simulink model "SWC_FDC_type"  (R2021b)
settings: Solver=FixedStepDiscrete  StartTime=0.0  StopTime=10.0  FixedStep=0.001  RelTol=1e-3
values from neighbouring files (symbols this model uses):
  DID_VCUKey = uint16(0x0202)    [vcu_local_hdr.m]
  DID_XWD = uint16(513)    [vcu_local_hdr.m]
  DIDLen_APSFunConfig = uint16(16)    [vcu_local_hdr.m]
  DIDLen_AutoLock = uint16(1)    [vcu_local_hdr.m]
  DIDLen_DKCKey = uint16(8)    [vcu_local_hdr.m]
  DIDLen_DRLDis = uint16(1)    [vcu_local_hdr.m]
  DIDLen_DynoMode = uint16(1)    [vcu_local_hdr.m]
  DIDLen_FMHTimer = uint16(1)    [vcu_local_hdr.m]
  DIDLen_LFLowPresThre = uint16(1)    [vcu_local_hdr.m]
  DIDLen_LFSensorID = uint16(4)    [vcu_local_hdr.m]
  DIDLen_LRLowPresThre = uint16(1)    [vcu_local_hdr.m]
  DIDLen_LRSensorID = uint16(4)    [vcu_local_hdr.m]
  DIDLen_RFLowPresThre = uint16(1)    [vcu_local_hdr.m]
  DIDLen_RFSensorID = uint16(4)    [vcu_local_hdr.m]
  DIDLen_RRLowPresThre = uint16(1)    [vcu_local_hdr.m]
  DIDLen_RRSensorID = uint16(4)    [vcu_local_hdr.m]
  DIDLen_SensorMode = uint16(1)    [vcu_local_hdr.m]
  DIDLen_TireSize = uint16(16)    [vcu_local_hdr.m]
  DIDLen_TPMSLearnSta = uint16(1)    [vcu_local_hdr.m]
  DIDLen_TurnLampFLThreCurr = uint16(1)    [vcu_local_hdr.m]
  DIDLen_TurnLampFRThreCurr = uint16(1)    [vcu_local_hdr.m]
  DIDLen_TurnLampRLThreCurr = uint16(1)    [vcu_local_hdr.m]
  DIDLen_TurnLampRRThreCurr = uint16(1)    [vcu_local_hdr.m]
  DIDLen_USSConfig = uint16(16)    [vcu_local_hdr.m]
  DIDLen_WhlPres = uint16(4)    [vcu_local_hdr.m]
  DIDLen_WhlSensorBattSta = uint16(1)    [vcu_local_hdr.m]
  DIDLen_WhlTmp = uint16(4)    [vcu_local_hdr.m]
  DIDLen_XWDMode = uint16(1)    [vcu_local_hdr.m]
  DIDNum_APSFunConfig = uint16(0x0903)    [vcu_local_hdr.m]
  DIDNum_AutoLock = uint16(0x0306)    [vcu_local_hdr.m]
  DIDNum_DKCKey = uint16(0x0202)    [vcu_local_hdr.m]
  DIDNum_DRLDis = uint16(0x0307)    [vcu_local_hdr.m]
  DIDNum_DynoMode = uint16(0x0203)    [vcu_local_hdr.m]
  DIDNum_FMHTimer = uint16(0x0305)    [vcu_local_hdr.m]
  DIDNum_LFLowPresThre = uint16(0x0B08)    [vcu_local_hdr.m]
  DIDNum_LFSensorID = uint16(0x0B01)    [vcu_local_hdr.m]
  DIDNum_LRLowPresThre = uint16(0x0B0A)    [vcu_local_hdr.m]
  DIDNum_LRSensorID = uint16(0x0B03)    [vcu_local_hdr.m]
  DIDNum_RFLowPresThre = uint16(0x0B09)    [vcu_local_hdr.m]
  DIDNum_RFSensorID = uint16(0x0B02)    [vcu_local_hdr.m]
  DIDNum_RRLowPresThre = uint16(0x0B0B)    [vcu_local_hdr.m]
  DIDNum_RRSensorID = uint16(0x0B04)    [vcu_local_hdr.m]
  DIDNum_SensorMode = uint16(0x0B0C)    [vcu_local_hdr.m]
  DIDNum_TireSize = uint16(0x0902)    [vcu_local_hdr.m]
  DIDNum_TPMSLearnSta = uint16(0x0B0D)    [vcu_local_hdr.m]
  DIDNum_TurnLampFLThreCurr = uint16(0x0303)    [vcu_local_hdr.m]
  DIDNum_TurnLampFRThreCurr = uint16(0x0301)    [vcu_local_hdr.m]
  DIDNum_TurnLampRLThreCurr = uint16(0x0304)    [vcu_local_hdr.m]
  DIDNum_TurnLampRRThreCurr = uint16(0x0302)    [vcu_local_hdr.m]
  DIDNum_USSConfig = uint16(0x0901)    [vcu_local_hdr.m]
  DIDNum_WhlPres = uint16(0x0B05)    [vcu_local_hdr.m]
  DIDNum_WhlSensorBattSta = uint16(0x0B07)    [vcu_local_hdr.m]
  DIDNum_WhlTmp = uint16(0x0B06)    [vcu_local_hdr.m]
  DIDNum_XWDMode = uint16(0x0201)    [vcu_local_hdr.m]
  DIDVCUKeyLength = uint16(8)    [vcu_local_hdr.m]
  ENUM_DRIVETRAIN_AWD = uint8(  2  )    [vcu_local_hdr.m]
  ENUM_DRIVETRAIN_FWD = uint8(  1  )    [vcu_local_hdr.m]
  ENUM_DRIVETRAIN_RWD = uint8(  0  )    [vcu_local_hdr.m]
  ENUM_REGENLEVEL_INVALID = uint8(  7  )    [vcu_local_hdr.m]
  ENUM_REGENLEVEL_LV1 = uint8(  1  )    [vcu_local_hdr.m]
  ENUM_REGENLEVEL_LV2 = uint8(  2  )    [vcu_local_hdr.m]
  ENUM_REGENLEVEL_LV3 = uint8(  3  )    [vcu_local_hdr.m]
  ENUM_REGENLEVEL_LV4 = uint8(  4  )    [vcu_local_hdr.m]
  ENUM_REGENLEVEL_LV5 = uint8(  5  )    [vcu_local_hdr.m]
  ENUM_REGENLEVEL_OFF = uint8(  0  )    [vcu_local_hdr.m]
  ENUM_REGENLEVEL_OPD = uint8(  6  )    [vcu_local_hdr.m]
  ENUM_TPMSLearnStatus_LEARNED = uint8(  1  )    [vcu_local_hdr.m]
  ENUM_TPMSLearnStatus_LEARNFAIL = uint8(  2  )    [vcu_local_hdr.m]
  ENUM_TPMSLearnStatus_NOTLEARN = uint8(  0  )    [vcu_local_hdr.m]
  ENUM_TPMSSTA_FAT = uint8(  8  )    [vcu_local_hdr.m]
  ENUM_TPMSSTA_LOWBATTERY = uint8(  2  )    [vcu_local_hdr.m]
  FALSE = boolean( 0 )    [vcu_local_hdr.m]
  ONE_INT = uint8(1)    [vcu_local_hdr.m]
  P_boolean = 0.0    [APPTypes.sldd]
  TRUE = boolean( 1 )    [vcu_local_hdr.m]
  ZERO_FLOAT = single(0)    [vcu_local_hdr.m]
  ZERO_INT = uint8(0)    [vcu_local_hdr.m]
undefined symbols (not defined in the file or in its folder): f32_ApsOutVehSpdSig, KHAL_DKCDecryptEnable_flg_ovrdflg, KHAL_DKCDecryptEnable_flg_ovrdval, KHAL_RandomNumberY1_enum, KHAL_RandomNumberY2_enum, KHAL_RandomNumberY_ovrdflg, KHAL_THCMAPTCWarningDTC_flg_ovrdflg, KHAL_THCMAPTCWarningDTC_flg_ovrdval, KHAL_TPMSRESBUTT_flg_ovrdflg, KHAL_TPMSRESBUTT_flg_ovrdval, R_DIDWriteCDD_CSOP_DIDSet_APSFunConfig, R_DIDWriteCDD_CSOP_DIDSet_AutoLock, R_DIDWriteCDD_CSOP_DIDSet_DKCKey, R_DIDWriteCDD_CSOP_DIDSet_DRLDis, R_DIDWriteCDD_CSOP_DIDSet_DynoMode, R_DIDWriteCDD_CSOP_DIDSet_FMHTimer, R_DIDWriteCDD_CSOP_DIDSet_LFLowPresThre, R_DIDWriteCDD_CSOP_DIDSet_LFSensorID, R_DIDWriteCDD_CSOP_DIDSet_LRLowPresThre, R_DIDWriteCDD_CSOP_DIDSet_LRSensorID, R_DIDWriteCDD_CSOP_DIDSet_RFLowPresThre, R_DIDWriteCDD_CSOP_DIDSet_RFSensorID, R_DIDWriteCDD_CSOP_DIDSet_RRLowPresThre, R_DIDWriteCDD_CSOP_DIDSet_RRSensorID, R_DIDWriteCDD_CSOP_DIDSet_SensorMode, R_DIDWriteCDD_CSOP_DIDSet_TireSize, R_DIDWriteCDD_CSOP_DIDSet_TPMSLearnSta, R_DIDWriteCDD_CSOP_DIDSet_TurnLampFLThreCurr, R_DIDWriteCDD_CSOP_DIDSet_TurnLampFRThreCurr, R_DIDWriteCDD_CSOP_DIDSet_TurnLampRLThreCurr, R_DIDWriteCDD_CSOP_DIDSet_TurnLampRRThreCurr, R_DIDWriteCDD_CSOP_DIDSet_USSConfig, R_DIDWriteCDD_CSOP_DIDSet_WhlPres, R_DIDWriteCDD_CSOP_DIDSet_WhlSensorBattSta, R_DIDWriteCDD_CSOP_DIDSet_WhlTmp, R_DIDWriteCDD_CSOP_DIDSet_XWDMode, R_E2E_CAN3_VCU1_CSOP_Write_CAN3_VCU1, R_E2E_CAN3_VCU1_toNIDEC_CSOP_Write_CAN3_VCU1_toNIDEC, R_E2E_CAN4_VCU1_CSOP_Write_CAN4_VCU1, R_FDCCDD_Inner_CSOP_FDC_AppCallSleep, R_HALINCDD_CSOP_PAS_Handler, R_HALINCDD_CSOP_UDS_Main, R_HALOUT_APS_CSOP_ApsOutput, R_HALOUTCDD_CSOP_AppNmStateReq, R_HALOUTCDD_CSOP_SetAcoreRebootCmdACK, R_HALOUTCDD_CSOP_SetSysPwrStat, R_HALOUTCDD_CSOP_SleepRequest, R_IOExpOUT_CDD_CSOP_IOExpSetVal, R_NVMReadCDD_Inner_NVM_ReadOperation, R_NVMWriteCDD_Inner_NVM_WriteOperation, R_UDSCDD_CSOP_DdmRestartOperationCycle, R_WDGCDD_CSOP_Call_Watchdog, R_WDGCDD_CSOP_Call_WDG_AppEnd, R_WDGCDD_CSOP_Call_WDG_AppStart, u16_DIDLen_APSFunConfig, u16_DIDLen_AutoLock, u16_DIDLen_DKCKey, u16_DIDLen_DRLDis, u16_DIDLen_DynoMode, u16_DIDLen_FMHTimer ... (+83)
libraries: simulink x215, FVT_lib x139, hcu_lib x21, hdlsllib x9, app x1, halin x1, halout x1, inp x1, outp x1
(part 11 of 12)

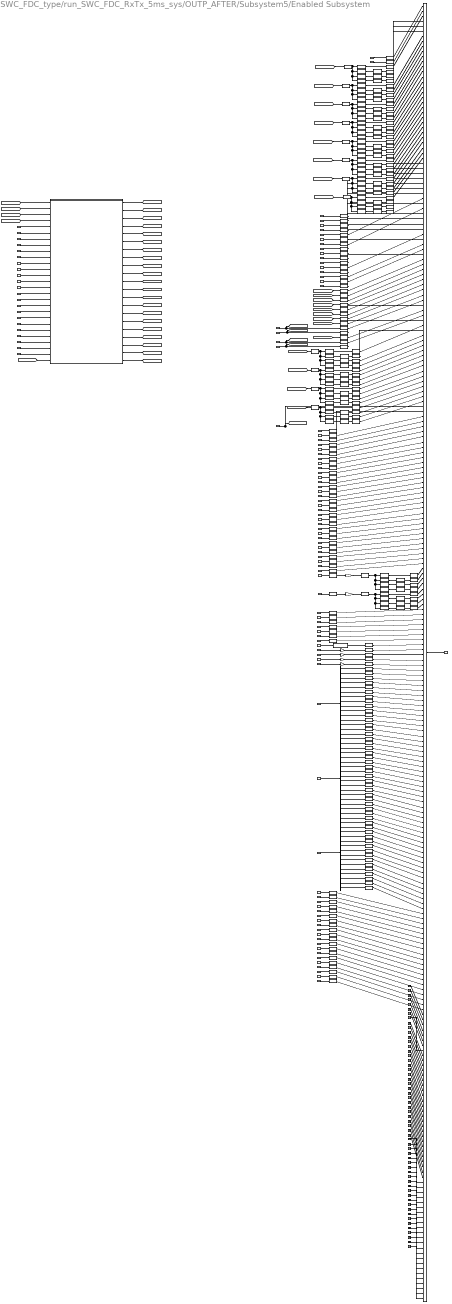
== system SWC_FDC_type/run_SWC_FDC_RxTx_5ms_sys/OUTP_AFTER/Subsystem5/Enabled Subsystem ==
  VOUTP_AntitheftSta_enum : Inport
  VOUTP_DrivetrainSelect_enum : Inport  Port=2
  VOUTP_WriteChkLFID_raw : Inport  Port=3
  VOUTP_WriteChkRFID_raw : Inport  Port=4
  VOUTP_WriteChkLRID_raw : Inport  Port=5
  VOUTP_WriteChkRRID_raw : Inport  Port=6
  VOUTP_WriteChkfinLFID_raw : Inport  Port=7
  VOUTP_WriteChkfinRFID_raw : Inport  Port=8
  VOUTP_WriteChkfinLRID_raw : Inport  Port=9
  VOUTP_WriteChkfinRRID_raw : Inport  Port=10
  VOUTP_LFSensorFail_flg : Inport  Port=11
  VOUTP_RFSensorFail_flg : Inport  Port=12
  VOUTP_LRSensorFail_flg : Inport  Port=13
  VOUTP_RRSensorFail_flg : Inport  Port=14
  VOUTP_LFWheelPSW_raw8 : Inport  Port=15
  VOUTP_RFWheelPSW_raw8 : Inport  Port=16
  VOUTP_LRWheelPSW_raw8 : Inport  Port=17
  VOUTP_RRWheelPSW_raw8 : Inport  Port=18
  VOUTP_LFPindi_enum : Inport  Port=19
  VOUTP_RFPindi_enum : Inport  Port=20
  VOUTP_LRPindi_enum : Inport  Port=21
  VOUTP_RRPindi_enum : Inport  Port=22
  VOUTP_LFP20_raw8 : Inport  Port=23
  VOUTP_RFP20_raw8 : Inport  Port=24
  VOUTP_LRP20_raw8 : Inport  Port=25
  VOUTP_RRP20_raw8 : Inport  Port=26
  VOUTP_LFWheelPress_raw8 : Inport  Port=27
  VOUTP_RFWheelPress_raw8 : Inport  Port=28
  VOUTP_LRWheelPress_raw8 : Inport  Port=29
  VOUTP_RRWheelPress_raw8 : Inport  Port=30
  VOUTP_LFWheelTemp_C : Inport  Port=31
  VOUTP_RFWheelTemp_C : Inport  Port=32
  VOUTP_LRWheelTemp_C : Inport  Port=33
  VOUTP_RRWheelTemp_C : Inport  Port=34
  VOUTP_Flashchkdatavalid_enum : Inport  Port=35
  VOUTP_Flashdatavalid_enum : Inport  Port=36
  VOUTP_unlearnSfali_flg : Inport  Port=37
  VOUTP_unlearnSfailvalid_enum : Inport  Port=38
  VOUTP_Prepresstempvalid_enum : Inport  Port=39
  VOUTP_FlashS1ID_raw : Inport  Port=40
  VOUTP_FlashS2ID_raw : Inport  Port=41
  VOUTP_FlashS3ID_raw : Inport  Port=42
  VOUTP_FlashS41ID_raw : Inport  Port=43
  VOUTP_FlashIDvalid_enum : Inport  Port=44
  VOUTP_ACModeMem_enum : Inport  Port=45
  VOUTP_Face_flg : Inport  Port=46
  VOUTP_Foot_flg : Inport  Port=47
  VOUTP_Frost_flg : Inport  Port=48
  VOUTP_FaceM_flg : Inport  Port=49
  VOUTP_FootM_flg : Inport  Port=50
  VOUTP_CCUSyncSts_flg : Inport  Port=51
  VOUTP_ACForceOFF_flg : Inport  Port=52
  VOUTP_sigRecircSt_flg : Inport  Port=53
  VOUTP_RecAutoFlg_flg : Inport  Port=54
  VOUTP_AirIntenZone1M_enum : Inport  Port=55
  VOUTP_fdefog_flg : Inport  Port=56
  VOUTP_sigSetTempZon1St_C : Inport  Port=57
  VOUTP_sigSetTempZon2StM_C : Inport  Port=58
  VOUT_CountAlarm_enum : Inport  Port=59
  VOUTP_MFSWTri_flg : Inport  Port=60
  VOUTP_MirrorFlodPos_flg : Inport  Port=61
  VOUTP_FuelDoorPos_flg : Inport  Port=62
  VOUTP_LockSetting_flg : Inport  Port=63
  VOUTP_MFRDNBrightReq_pct : Inport  Port=64
  VOUTP_RoomLampMode_flg : Inport  Port=65
  VOUTP_WiperFixMode_flg : Inport  Port=66
  VOUTP_IVIPTGUSStaSW_flg : Inport  Port=67
  VOUTP_EAPS1MIN_pct : Inport  Port=68
  VOUTP_EAPS2MIN_pct : Inport  Port=69
  VOUTP_HoodSW_flg : Inport  Port=70
  VOUTP_TailgateSW_flg : Inport  Port=71
  VOUTP_CTDLockSW_flg : Inport  Port=72
  VOUTP_TailgateHDSW_flg : Inport  Port=73
  VOUTP_APMDoorControlSta_flg : Inport  Port=74
  VOUTP_fUnlockSingle_flg : Inport  Port=75
  VOUTP_SaveRegenMode_enum : Inport  Port=76
  VOUTP_AmbFunENFlash_enum : Inport  Port=77
  VOUTP_AmbWelENFlash_enum : Inport  Port=78
  VOUTP_AmbDimENFlash_enum : Inport  Port=79
  VOUTP_AmbLinkDriStaFlash_enum : Inport  Port=80
  VOUTP_AmbPwrWarnENFlash_enum : Inport  Port=81
  VOUTP_AmbODAENFlash_enum : Inport  Port=82
  VOUTP_AmbColorSta1_enum : Inport  Port=83
  VOUTP_AmbColorSta2_enum : Inport  Port=84
  VOUTP_AmbColorSta3_enum : Inport  Port=85
  VOUTP_AmbColorSta4_enum : Inport  Port=86
  VOUTP_AmbColorSta5_enum : Inport  Port=87
  VOUTP_AmbColorSta7_enum : Inport  Port=88
  VOUTP_AmbBrightnessSta1_enum : Inport  Port=89
  VOUTP_AmbBrightnessSta2_enum : Inport  Port=90
  VOUTP_AmbBrightnessSta3_enum : Inport  Port=91
  VOUTP_AmbBrightnessSta4_enum : Inport  Port=92
  VOUTP_AmbBrightnessSta5_enum : Inport  Port=93
  VOUTP_AmbBrightnessSta7_enum : Inport  Port=94
  BHAL_SYSTPMS_outputs : Inport  Port=95
  VHAL_RandomnumberY_raw1 : Inport  Port=96
  VHAL_RandomnumberY_raw2 : Inport  Port=97
  VHAL_RandomnumberY_raw3 : Inport  Port=98
  VHAL_RandomnumberY_raw4 : Inport  Port=99
  VHAL_RandomnumberY_raw5 : Inport  Port=100
  VHAL_RandomnumberY_raw6 : Inport  Port=101
  VHAL_RandomnumberY_raw7 : Inport  Port=102
  VHAL_RandomnumberY_raw8 : Inport  Port=103
  VHAL_funAuto_flg : Inport  Port=104
  VHAL_DiagDRLOFF_flg : Inport  Port=105
  VHAL_DiagFMHT_s : Inport  Port=106
  VHAL_DiagFLTC_mA : Inport  Port=107
  VHAL_DiagFRTC_mA : Inport  Port=108
  VHAL_DiagRLTC_mA : Inport  Port=109
  VHAL_DiagRRTC_mA : Inport  Port=110
  VHAL_USSConfig_raw8 : Inport  Port=111
  VHAL_TireSize_raw8 : Inport  Port=112
  VHAL_APSFunConfig_raw8 : Inport  Port=113
  Bitwise AND{,4,8,14,16,22,26,30,32,36,40,44,48,52} (14 alike) : simulink/Logic and Bit Operations/Bitwise Operator  logicop=AND  UseBitMask=on  BitMask=bin2dec('00000000000000000000000011111111')  BitMaskRealWorld=Stored Integer
  Bitwise AND{1,5,9,15,17,23,27,31,33,37,41,45,49,53} (14 alike) : simulink/Logic and Bit Operations/Bitwise Operator  logicop=AND  UseBitMask=on  BitMask=bin2dec('00000000000000001111111100000000')  BitMaskRealWorld=Stored Integer
  Bitwise AND{2,6,10,12,18,20,24,28,34,38,42,46,50,54} (14 alike) : simulink/Logic and Bit Operations/Bitwise Operator  logicop=AND  UseBitMask=on  BitMask=bin2dec('00000000111111110000000000000000')  BitMaskRealWorld=Stored Integer
  Bitwise AND{3,7,11,13,19,21,25,29,35,39,43,47,51,55} (14 alike) : simulink/Logic and Bit Operations/Bitwise Operator  logicop=AND  UseBitMask=on  BitMask=bin2dec('11111111000000000000000000000000')  BitMaskRealWorld=Stored Integer
  Data Type Conversion{,1,5..13,15..18,20..23,25..27,29..32,34..37,39..40,42..106,108..111,113..116,118..121,123..126,128..130,132..213} (198 alike) : DataTypeConversion  OutDataTypeStr=uint8
  Data Type Conversion{4,14,19,24,28,33,38,41,107,112,117,122,127,131} (14 alike) : DataTypeConversion  OutDataTypeStr=uint32
  Data Type Conversion2 : DataTypeConversion  OutDataTypeStr=single
  Data Type Conversion3 : DataTypeConversion  OutDataTypeStr=single
  Demux : Demux  Outputs=16
  Demux1 : Demux  Outputs=16
  Demux2 : Demux  Outputs=16
  Gain{,1..3} (4 alike) : Gain  Gain=1/10
  Ground{183..187,196..198,200..247,251} (57 alike) : Ground
  Multiply : Gain  Gain=10000
  Multiply1 : Gain  Gain=10000
  Mux : Mux  Inputs=256
  NVM1 : Subsystem
  Shift Arithmetic{,3,6,9,12,17,20,23..24,27,30,33,36,39} (14 alike) : ArithShift  BitShiftNumber=8  BitShiftDirection=Right
  Shift Arithmetic{1,4,7,10,13..14,18,21,25,28,31,34,37,40} (14 alike) : ArithShift  BitShiftNumber=16  BitShiftDirection=Right
  Shift Arithmetic{2,5,8,11,15..16,19,22,26,29,32,35,38,41} (14 alike) : ArithShift  BitShiftNumber=24  BitShiftDirection=Right
  Subsystem : Subsystem
  HAL_NvmWriteData_raw : Outport
  wires:
  Bitwise AND20/1 -> Shift Arithmetic14/1
  Shift Arithmetic4/1 -> Data Type Conversion12/1
  Data Type Conversion12/1 -> Mux/9
  Data Type Conversion30/1 -> Mux/24
  Shift Arithmetic23/1 -> Data Type Conversion40/1
  Bitwise AND1/1 -> Shift Arithmetic/1
  Bitwise AND11/1 -> Shift Arithmetic8/1
  Data Type Conversion5/1 -> Mux/21
  Bitwise AND17/1 -> Shift Arithmetic12/1
  Data Type Conversion32/1 -> Mux/30
  Data Type Conversion13/1 -> Mux/10
  Shift Arithmetic22/1 -> Data Type Conversion32/1
  Shift Arithmetic17/1 -> Data Type Conversion30/1
  Shift Arithmetic18/1 -> Data Type Conversion7/1
  Data Type Conversion14/1 -> Bitwise AND4/1, Bitwise AND7/1, Bitwise AND6/1, Bitwise AND5/1
  Bitwise AND26/1 -> Data Type Conversion29/1
  Data Type Conversion17/1 -> Mux/13
  Data Type Conversion25/1 -> Mux/15
  Data Type Conversion18/1 -> Mux/14
  Bitwise AND29/1 -> Shift Arithmetic19/1
  Shift Arithmetic8/1 -> Data Type Conversion18/1
  Data Type Conversion39/1 -> Mux/31
  Shift Arithmetic10/1 -> Data Type Conversion22/1
  Data Type Conversion6/1 -> Mux/22
  Bitwise AND28/1 -> Shift Arithmetic18/1
  Shift Arithmetic/1 -> Data Type Conversion9/1
  Data Type Conversion42/1 -> Mux/19
  Data Type Conversion11/1 -> Mux/6
  Shift Arithmetic19/1 -> Data Type Conversion27/1
  Data Type Conversion28/1 -> Bitwise AND26/1, Bitwise AND27/1, Bitwise AND28/1, Bitwise AND29/1
  Bitwise AND19/1 -> Shift Arithmetic22/1
  Bitwise AND27/1 -> Shift Arithmetic17/1
  Bitwise AND3/1 -> Shift Arithmetic2/1
  Data Type Conversion1/1 -> Mux/2
  Data Type Conversion26/1 -> Mux/16
  Bitwise AND23/1 -> Shift Arithmetic23/1
  Shift Arithmetic7/1 -> Data Type Conversion17/1
  Shift Arithmetic21/1 -> Data Type Conversion31/1
  Data Type Conversion8/1 -> Mux/3
  Data Type Conversion/1 -> Mux/1
  Bitwise AND10/1 -> Shift Arithmetic7/1
  Data Type Conversion37/1 -> Mux/34
  Data Type Conversion40/1 -> Mux/32
  Data Type Conversion36/1 -> Mux/33
  Bitwise AND/1 -> Data Type Conversion8/1
  Data Type Conversion20/1 -> Mux/11
  Data Type Conversion16/1 -> Mux/8
  Data Type Conversion21/1 -> Mux/12
  Data Type Conversion9/1 -> Mux/4
  Data Type Conversion10/1 -> Mux/5
  Data Type Conversion31/1 -> Mux/29
  Data Type Conversion15/1 -> Mux/7
  Data Type Conversion34/1 -> Mux/27
  Data Type Conversion35/1 -> Mux/28
  Data Type Conversion27/1 -> Mux/26
  Data Type Conversion29/1 -> Mux/23
  Data Type Conversion7/1 -> Mux/25
  Data Type Conversion22/1 -> Mux/17
  Data Type Conversion23/1 -> Mux/18
  Data Type Conversion43/1 -> Mux/20
  Data Type Conversion33/1 -> Bitwise AND19/1, Bitwise AND18/1, Bitwise AND31/1, Bitwise AND30/1
  Data Type Conversion41/1 -> Bitwise AND25/1, Bitwise AND24/1, Bitwise AND17/1, Bitwise AND16/1
  Bitwise AND30/1 -> Data Type Conversion34/1
  Bitwise AND24/1 -> Shift Arithmetic13/1
  Shift Arithmetic12/1 -> Data Type Conversion43/1
  Bitwise AND25/1 -> Shift Arithmetic16/1
  Bitwise AND18/1 -> Shift Arithmetic21/1
  Shift Arithmetic16/1 -> Data Type Conversion6/1
  Shift Arithmetic15/1 -> Data Type Conversion37/1
  Data Type Conversion38/1 -> Bitwise AND21/1, Bitwise AND20/1, Bitwise AND23/1, Bitwise AND22/1
  Bitwise AND31/1 -> Shift Arithmetic20/1
  Shift Arithmetic9/1 -> Data Type Conversion26/1
  Bitwise AND21/1 -> Shift Arithmetic15/1
  Data Type Conversion24/1 -> Bitwise AND14/1, Bitwise AND13/1, Bitwise AND12/1, Bitwise AND15/1
  Bitwise AND13/1 -> Shift Arithmetic11/1
  Bitwise AND9/1 -> Shift Arithmetic6/1
  Bitwise AND15/1 -> Shift Arithmetic9/1
  Bitwise AND12/1 -> Shift Arithmetic10/1
  Bitwise AND7/1 -> Shift Arithmetic5/1
  Shift Arithmetic2/1 -> Data Type Conversion11/1
  Shift Arithmetic1/1 -> Data Type Conversion10/1
  Data Type Conversion19/1 -> Bitwise AND11/1, Bitwise AND10/1, Bitwise AND9/1, Bitwise AND8/1
  Bitwise AND6/1 -> Shift Arithmetic4/1
  Bitwise AND5/1 -> Shift Arithmetic3/1
  Shift Arithmetic20/1 -> Data Type Conversion35/1
  Shift Arithmetic5/1 -> Data Type Conversion13/1
  Bitwise AND4/1 -> Data Type Conversion15/1
  Shift Arithmetic3/1 -> Data Type Conversion16/1
  Bitwise AND8/1 -> Data Type Conversion20/1
  Bitwise AND22/1 -> Data Type Conversion39/1
  Data Type Conversion4/1 -> Bitwise AND3/1, Bitwise AND2/1, Bitwise AND1/1, Bitwise AND/1
  Bitwise AND2/1 -> Shift Arithmetic1/1
  Shift Arithmetic11/1 -> Data Type Conversion23/1
  Shift Arithmetic14/1 -> Data Type Conversion36/1
  Shift Arithmetic13/1 -> Data Type Conversion5/1
  Bitwise AND14/1 -> Data Type Conversion25/1
  Shift Arithmetic6/1 -> Data Type Conversion21/1
  Bitwise AND16/1 -> Data Type Conversion42/1
  VOUTP_DrivetrainSelect_enum/1 -> Data Type Conversion1/1
  VOUTP_AntitheftSta_enum/1 -> Data Type Conversion/1
  Data Type Conversion66/1 -> Mux/57
  Data Type Conversion67/1 -> Mux/55
  VOUTP_ACModeMem_enum/1 -> Data Type Conversion81/1
  Data Type Conversion57/1 -> Mux/48
  VHAL_RandomnumberY_raw7/1 -> Data Type Conversion79/1
  VHAL_RandomnumberY_raw5/1 -> Data Type Conversion77/1
  VHAL_RandomnumberY_raw6/1 -> Data Type Conversion78/1
  Data Type Conversion72/1 -> Mux/62
  Data Type Conversion69/1 -> Mux/59
  VOUTP_Foot_flg/1 -> Data Type Conversion83/1
  [VHAL_NVMLRWheelPress_raw8] -> Data Type Conversion62/1
  VOUTP_LFSensorFail_flg/1 -> Data Type Conversion47/1
  [VHAL_NVMLFWheelPress_raw8] -> Data Type Conversion63/1
  VHAL_RandomnumberY_raw4/1 -> Data Type Conversion76/1
  VOUTP_Flashchkdatavalid_enum/1 -> [VOUTP_Flashchkdatavalid_enum], Data Type Conversion69/1
  Data Type Conversion63/1 -> Mux/51
  Data Type Conversion68/1 -> Mux/58
  Data Type Conversion51/1 -> Mux/39
  Data Type Conversion53/1 -> Mux/44
  VHAL_RandomnumberY_raw1/1 -> Data Type Conversion75/1
  Data Type Conversion48/1 -> Mux/38
  VOUTP_Face_flg/1 -> Data Type Conversion82/1
  VOUTP_LFP20_raw8/1 -> Data Type Conversion59/1
  VOUTP_CCUSyncSts_flg/1 -> Data Type Conversion87/1
  VHAL_RandomnumberY_raw3/1 -> Data Type Conversion74/1
  [VHAL_NVMRFWheelPress_raw8] -> Data Type Conversion61/1
  Data Type Conversion54/1 -> Mux/45
  Data Type Conversion47/1 -> Mux/35
  [VHAL_NVMunlearnSfali_flg] -> Data Type Conversion71/1
  VOUTP_RecAutoFlg_flg/1 -> Data Type Conversion90/1
  Data Type Conversion61/1 -> Mux/52
  VOUTP_fdefog_flg/1 -> Data Type Conversion92/1
  Data Type Conversion55/1 -> Mux/43
  VOUTP_sigRecircSt_flg/1 -> Data Type Conversion89/1
  Data Type Conversion52/1 -> Mux/42
  Data Type Conversion93/1 -> Mux/63
  Data Type Conversion56/1 -> Mux/46
  VOUTP_RFP20_raw8/1 -> Data Type Conversion57/1
  VOUTP_Prepresstempvalid_enum/1 -> [VOUTP_Prepresstempvalid_enum], Data Type Conversion93/1
  VOUTP_FaceM_flg/1 -> Data Type Conversion85/1
  Data Type Conversion58/1 -> Mux/49
  Data Type Conversion65/1 -> Mux/56
  VOUTP_RRPindi_enum/1 -> Data Type Conversion56/1
  VOUTP_FootM_flg/1 -> Data Type Conversion86/1
  Data Type Conversion50/1 -> Mux/41
  VOUTP_Flashdatavalid_enum/1 -> [VOUTP_Flashdatavalid_enum], Data Type Conversion70/1
  [VHAL_NVMRRWheelPress_raw8] -> Data Type Conversion64/1
  Data Type Conversion70/1 -> Mux/60
  [VHAL_NVMRRWheelTemp_C] -> Data Type Conversion68/1
  [VHAL_NVMLFWheelTemp_C] -> Data Type Conversion67/1
  VOUTP_AirIntenZone1M_enum/1 -> Data Type Conversion91/1
  Data Type Conversion64/1 -> Mux/54
  VOUTP_LRP20_raw8/1 -> Data Type Conversion58/1
  Data Type Conversion71/1 -> Mux/61
  VOUTP_RFPindi_enum/1 -> Data Type Conversion53/1
  VOUTP_RRP20_raw8/1 -> Data Type Conversion60/1
  Data Type Conversion49/1 -> Mux/40
  VOUTP_LRPindi_enum/1 -> Data Type Conversion54/1
  VOUTP_LFPindi_enum/1 -> Data Type Conversion55/1
  [VHAL_NVMLRWheelTemp_C] -> Data Type Conversion66/1
  Data Type Conversion62/1 -> Mux/53
  Data Type Conversion60/1 -> Mux/50
  Data Type Conversion59/1 -> Mux/47
  VOUTP_RRWheelPSW_raw8/1 -> Data Type Conversion52/1
  VHAL_RandomnumberY_raw2/1 -> Data Type Conversion73/1
  VOUTP_LRWheelPSW_raw8/1 -> Data Type Conversion50/1
  VHAL_RandomnumberY_raw8/1 -> Data Type Conversion80/1
  Data Type Conversion45/1 -> Mux/36
  VOUTP_ACForceOFF_flg/1 -> Data Type Conversion88/1
  Data Type Conversion46/1 -> Mux/37
  VOUTP_LFWheelPSW_raw8/1 -> Data Type Conversion51/1
  VOUTP_RRSensorFail_flg/1 -> Data Type Conversion48/1
  VOUTP_LRSensorFail_flg/1 -> Data Type Conversion46/1
  [VHAL_NVMRFWheelTemp_C] -> Data Type Conversion65/1
  VOUTP_RFWheelPSW_raw8/1 -> Data Type Conversion49/1
  VOUTP_RFSensorFail_flg/1 -> Data Type Conversion45/1
  VOUTP_Frost_flg/1 -> Data Type Conversion84/1
  Data Type Conversion134/1 -> Mux/120
  Data Type Conversion135/1 -> Mux/121
  Data Type Conversion136/1 -> Mux/122
  Data Type Conversion137/1 -> Mux/123
  Ground185/1 -> Mux/202
  Ground183/1 -> Mux/200
  Ground184/1 -> Mux/201
  Ground197/1 -> Mux/206
  Ground196/1 -> Mux/205
  Ground187/1 -> Mux/204
  Ground186/1 -> Mux/203
  Ground198/1 -> Mux/207
  Ground211/1 -> Mux/228
  Ground221/1 -> Mux/224
  Ground208/1 -> Mux/225
  Ground220/1 -> Mux/223
  Ground218/1 -> Mux/221
  Ground209/1 -> Mux/226
  Ground216/1 -> Mux/219
  Ground217/1 -> Mux/220
  Ground205/1 -> Mux/214
  Ground215/1 -> Mux/218
  Ground207/1 -> Mux/216
  Ground204/1 -> Mux/213
  Ground206/1 -> Mux/215
  Ground203/1 -> Mux/212
  Ground202/1 -> Mux/211
  Ground200/1 -> Mux/209
  Ground201/1 -> Mux/210
  Ground210/1 -> Mux/227
  Ground225/1 -> Mux/208
  Ground214/1 -> Mux/217
  Ground223/1 -> Mux/232
  Ground222/1 -> Mux/231
  Ground213/1 -> Mux/230
  Ground212/1 -> Mux/229
  Ground224/1 -> Mux/233
  Ground219/1 -> Mux/222
  Ground237/1 -> Mux/254
  Ground247/1 -> Mux/250
  Ground234/1 -> Mux/251
  Ground246/1 -> Mux/249
  Ground244/1 -> Mux/247
  Ground235/1 -> Mux/252
  Ground242/1 -> Mux/245
  Ground243/1 -> Mux/246
  Ground231/1 -> Mux/240
  Ground241/1 -> Mux/244
  Ground233/1 -> Mux/242
  Ground230/1 -> Mux/239
  Ground232/1 -> Mux/241
  Ground229/1 -> Mux/238
  Ground228/1 -> Mux/237
  Ground226/1 -> Mux/235
  Ground227/1 -> Mux/236
  Ground236/1 -> Mux/253
  Ground251/1 -> Mux/234
  Ground240/1 -> Mux/243
  Ground239/1 -> Mux/256
  Ground238/1 -> Mux/255
  Ground245/1 -> Mux/248
  Mux/1 -> HAL_NvmWriteData_raw/1
  NVM1/1(VHAL_NVMWriteChkLFID_raw) -> [VHAL_NVMWriteChkLFID_raw]
  VOUTP_WriteChkRFID_raw/1 -> NVM1/6(VOUTP_WriteChkRFID_raw)
  VOUTP_WriteChkLFID_raw/1 -> NVM1/5(VOUTP_WriteChkLFID_raw)
  VOUTP_WriteChkRRID_raw/1 -> NVM1/8(VOUTP_WriteChkRRID_raw)
  VOUTP_WriteChkLRID_raw/1 -> NVM1/7(VOUTP_WriteChkLRID_raw)
  [VOUTP_unlearnSfailvalid_enum] -> NVM1/3(VOUTP_unlearnSfailvalid_enum)
  [VOUTP_Flashchkdatavalid_enum] -> NVM1/1(VOUTP_Flashchkdatavalid_enum)
  [VOUTP_Prepresstempvalid_enum] -> NVM1/4(VOUTP_Prepresstempvalid_enum)
  [VOUTP_Flashdatavalid_enum] -> NVM1/2(VOUTP_Flashdatavalid_enum)
  VOUTP_unlearnSfailvalid_enum/1 -> Data Type Conversion72/1, [VOUTP_unlearnSfailvalid_enum]
  [VHAL_NVMWriteChkfinRRID_raw] -> Data Type Conversion38/1
  [VHAL_NVMWriteChkfinLRID_raw] -> Data Type Conversion33/1
  [VHAL_NVMWriteChkfinRFID_raw] -> Data Type Conversion28/1
  [VHAL_NVMWriteChkfinLFID_raw] -> Data Type Conversion41/1
  [VHAL_NVMWriteChkRRID_raw] -> Data Type Conversion24/1
  [VHAL_NVMWriteChkLRID_raw] -> Data Type Conversion19/1
  [VHAL_NVMWriteChkRFID_raw] -> Data Type Conversion14/1
  [VHAL_NVMWriteChkLFID_raw] -> Data Type Conversion4/1
  VOUT_CountAlarm_enum/1 -> Data Type Conversion99/1
  VOUTP_FuelDoorPos_flg/1 -> Data Type Conversion96/1
  VOUTP_LockSetting_flg/1 -> Data Type Conversion103/1
  VOUTP_WiperFixMode_flg/1 -> Data Type Conversion104/1
  VOUTP_MFRDNBrightReq_pct/1 -> Data Type Conversion100/1
  VOUTP_IVIPTGUSStaSW_flg/1 -> Data Type Conversion102/1
  VOUTP_RoomLampMode_flg/1 -> Data Type Conversion101/1
  VOUTP_MirrorFlodPos_flg/1 -> Data Type Conversion95/1
  VOUTP_sigSetTempZon2StM_C/1 -> Data Type Conversion98/1
  VOUTP_sigSetTempZon1St_C/1 -> Data Type Conversion97/1
  VOUTP_MFSWTri_flg/1 -> Data Type Conversion94/1
  VOUTP_WriteChkfinLRID_raw/1 -> NVM1/11(VOUTP_WriteChkfinLRID_raw)
  VOUTP_WriteChkfinRRID_raw/1 -> NVM1/12(VOUTP_WriteChkfinRRID_raw)
  VOUTP_WriteChkfinLFID_raw/1 -> NVM1/9(VOUTP_WriteChkfinLFID_raw)
  VOUTP_WriteChkfinRFID_raw/1 -> NVM1/10(VOUTP_WriteChkfinRFID_raw)
  VOUTP_LFWheelPress_raw8/1 -> NVM1/13(VOUTP_LFWheelPress_raw8)
  VOUTP_RFWheelPress_raw8/1 -> NVM1/14(VOUTP_RFWheelPress_raw8)
  VOUTP_RRWheelPress_raw8/1 -> NVM1/16(VOUTP_RRWheelPress_raw8)
  VOUTP_LRWheelPress_raw8/1 -> NVM1/15(VOUTP_LRWheelPress_raw8)
  VOUTP_LFWheelTemp_C/1 -> NVM1/17(VOUTP_LFWheelTemp_C)
  VOUTP_RFWheelTemp_C/1 -> NVM1/18(VOUTP_RFWheelTemp_C)
  VOUTP_LRWheelTemp_C/1 -> NVM1/19(VOUTP_LRWheelTemp_C)
  VOUTP_RRWheelTemp_C/1 -> NVM1/20(VOUTP_RRWheelTemp_C)
  VOUTP_unlearnSfali_flg/1 -> NVM1/21(VOUTP_unlearnSfali_flg)
  BHAL_SYSTPMS_outputs/1 -> NVM1/22(BHAL_SYSTPMS_outputs)
  VOUTP_FlashS41ID_raw/1 -> NVM1/26(VOUTP_FlashS4ID_raw)
  VOUTP_FlashS2ID_raw/1 -> NVM1/24(VOUTP_FlashS2ID_raw)
  VOUTP_FlashS1ID_raw/1 -> NVM1/23(VOUTP_FlashS1ID_raw)
  VOUTP_FlashS3ID_raw/1 -> NVM1/25(VOUTP_FlashS3ID_raw)
  [VOUTP_FlashIDvalid_enum] -> NVM1/27(VOUTP_FlashIDvalid_enum)
  VOUTP_FlashIDvalid_enum/1 -> Mux/80, [VOUTP_FlashIDvalid_enum]
  Shift Arithmetic32/1 -> Data Type Conversion116/1
  Bitwise AND35/1 -> Shift Arithmetic26/1
  Shift Arithmetic29/1 -> Data Type Conversion111/1
  Bitwise AND43/1 -> Shift Arithmetic32/1
  Bitwise AND33/1 -> Shift Arithmetic24/1
  Bitwise AND41/1 -> Shift Arithmetic30/1
  [VHAL_NVMFlashS4ID_raw] -> Data Type Conversion122/1
  Shift Arithmetic24/1 -> Data Type Conversion109/1
  Data Type Conversion107/1 -> Bitwise AND35/1, Bitwise AND34/1, Bitwise AND33/1, Bitwise AND32/1
  Shift Arithmetic33/1 -> Data Type Conversion124/1
  Shift Arithmetic34/1 -> Data Type Conversion120/1
  Data Type Conversion117/1 -> Bitwise AND43/1, Bitwise AND42/1, Bitwise AND41/1, Bitwise AND40/1
  Bitwise AND36/1 -> Data Type Conversion113/1
  Bitwise AND40/1 -> Data Type Conversion118/1
  Shift Arithmetic27/1 -> Data Type Conversion114/1
  Bitwise AND32/1 -> Data Type Conversion108/1
  Bitwise AND37/1 -> Shift Arithmetic27/1
  Data Type Conversion122/1 -> Bitwise AND47/1, Bitwise AND46/1, Bitwise AND45/1, Bitwise AND44/1
  Shift Arithmetic26/1 -> Data Type Conversion106/1
  Data Type Conversion112/1 -> Bitwise AND39/1, Bitwise AND38/1, Bitwise AND37/1, Bitwise AND36/1
  Bitwise AND39/1 -> Shift Arithmetic29/1
  Bitwise AND47/1 -> Shift Arithmetic35/1
  Bitwise AND44/1 -> Data Type Conversion123/1
  Bitwise AND46/1 -> Shift Arithmetic34/1
  [VHAL_NVMFlashS3ID_raw] -> Data Type Conversion117/1
  Shift Arithmetic30/1 -> Data Type Conversion119/1
  Bitwise AND34/1 -> Shift Arithmetic25/1
  Shift Arithmetic28/1 -> Data Type Conversion110/1
  Bitwise AND38/1 -> Shift Arithmetic28/1
  Bitwise AND45/1 -> Shift Arithmetic33/1
  [VHAL_NVMFlashS2ID_raw] -> Data Type Conversion112/1
  Shift Arithmetic25/1 -> Data Type Conversion105/1
  Shift Arithmetic35/1 -> Data Type Conversion121/1
  Shift Arithmetic31/1 -> Data Type Conversion115/1
  Bitwise AND42/1 -> Shift Arithmetic31/1
  [VHAL_NVMFlashS1ID_raw] -> Data Type Conversion107/1
  Data Type Conversion109/1 -> Mux/65
  Data Type Conversion105/1 -> Mux/66
  Data Type Conversion106/1 -> Mux/67
  Data Type Conversion114/1 -> Mux/69
  Data Type Conversion110/1 -> Mux/70
  Data Type Conversion111/1 -> Mux/71
  Data Type Conversion119/1 -> Mux/73
  Data Type Conversion115/1 -> Mux/74
  Data Type Conversion116/1 -> Mux/75
  Data Type Conversion124/1 -> Mux/77
  Data Type Conversion120/1 -> Mux/78
  Data Type Conversion121/1 -> Mux/79
  Data Type Conversion108/1 -> Mux/64
  Data Type Conversion113/1 -> Mux/68
  Data Type Conversion118/1 -> Mux/72
  Data Type Conversion123/1 -> Mux/76
  Data Type Conversion75/1 -> Mux/81
  Data Type Conversion73/1 -> Mux/82
  Data Type Conversion74/1 -> Mux/83
  Data Type Conversion76/1 -> Mux/84
  Data Type Conversion77/1 -> Mux/85
  Data Type Conversion78/1 -> Mux/86
  Data Type Conversion79/1 -> Mux/87
  Data Type Conversion80/1 -> Mux/88
  Data Type Conversion81/1 -> Mux/89
  Data Type Conversion82/1 -> Mux/90
  Data Type Conversion83/1 -> Mux/91
  Data Type Conversion84/1 -> Mux/92
  Data Type Conversion85/1 -> Mux/93
  Data Type Conversion86/1 -> Mux/94
  Data Type Conversion87/1 -> Mux/95
  Data Type Conversion88/1 -> Mux/96
  Data Type Conversion89/1 -> Mux/97
  Data Type Conversion90/1 -> Mux/98
  Data Type Conversion91/1 -> Mux/99
  Data Type Conversion92/1 -> Mux/100
  Data Type Conversion97/1 -> Mux/101
  Data Type Conversion98/1 -> Mux/102
  Data Type Conversion99/1 -> Mux/103
  Data Type Conversion94/1 -> Mux/104
  Data Type Conversion95/1 -> Mux/105
  Data Type Conversion96/1 -> Mux/106
  Data Type Conversion103/1 -> Mux/107
  Data Type Conversion100/1 -> Mux/108
  Data Type Conversion101/1 -> Mux/109
  Data Type Conversion104/1 -> Mux/110
  Data Type Conversion102/1 -> Mux/111
  NVM1/21(VHAL_NVMFlashS4ID_raw) -> [VHAL_NVMFlashS4ID_raw]
  NVM1/2(VHAL_NVMWriteChkRFID_raw) -> [VHAL_NVMWriteChkRFID_raw]
  NVM1/3(VHAL_NVMWriteChkLRID_raw) -> [VHAL_NVMWriteChkLRID_raw]
  NVM1/4(VHAL_NVMWriteChkRRID_raw) -> [VHAL_NVMWriteChkRRID_raw]
  NVM1/5(VHAL_NVMWriteChkfinLFID_raw) -> [VHAL_NVMWriteChkfinLFID_raw]
  NVM1/6(VHAL_NVMWriteChkfinRFID_raw) -> [VHAL_NVMWriteChkfinRFID_raw]
  NVM1/7(VHAL_NVMWriteChkfinLRID_raw) -> [VHAL_NVMWriteChkfinLRID_raw]
  NVM1/8(VHAL_NVMWriteChkfinRRID_raw) -> [VHAL_NVMWriteChkfinRRID_raw]
  NVM1/9(VHAL_NVMunlearnSfali_flg) -> [VHAL_NVMunlearnSfali_flg]
  NVM1/10(VHAL_NVMLFWheelPress_raw8) -> [VHAL_NVMLFWheelPress_raw8]
  NVM1/11(VHAL_NVMRFWheelPress_raw8) -> [VHAL_NVMRFWheelPress_raw8]
  NVM1/12(VHAL_NVMLRWheelPress_raw8) -> [VHAL_NVMLRWheelPress_raw8]
  NVM1/13(VHAL_NVMRRWheelPress_raw8) -> [VHAL_NVMRRWheelPress_raw8]
  NVM1/14(VHAL_NVMLFWheelTemp_C) -> [VHAL_NVMLFWheelTemp_C]
  NVM1/15(VHAL_NVMRFWheelTemp_C) -> [VHAL_NVMRFWheelTemp_C]
  NVM1/16(VHAL_NVMLRWheelTemp_C) -> [VHAL_NVMLRWheelTemp_C]
  NVM1/17(VHAL_NVMRRWheelTemp_C) -> [VHAL_NVMRRWheelTemp_C]
  NVM1/18(VHAL_NVMFlashS1ID_raw) -> [VHAL_NVMFlashS1ID_raw]
  NVM1/19(VHAL_NVMFlashS2ID_raw) -> [VHAL_NVMFlashS2ID_raw]
  NVM1/20(VHAL_NVMFlashS3ID_raw) -> [VHAL_NVMFlashS3ID_raw]
  VOUTP_EAPS1MIN_pct/1 -> Data Type Conversion2/1
  VOUTP_EAPS2MIN_pct/1 -> Data Type Conversion3/1
  Multiply/1 -> Data Type Conversion127/1
  Data Type Conversion126/1 -> Mux/115
  Data Type Conversion129/1 -> Mux/113
  Data Type Conversion125/1 -> Mux/114
  Shift Arithmetic37/1 -> Data Type Conversion125/1
  Shift Arithmetic38/1 -> Data Type Conversion126/1
  Data Type Conversion128/1 -> Mux/112
  Bitwise AND48/1 -> Data Type Conversion128/1
  Bitwise AND49/1 -> Shift Arithmetic36/1
  Data Type Conversion127/1 -> Bitwise AND51/1, Bitwise AND50/1, Bitwise AND49/1, Bitwise AND48/1
  Shift Arithmetic36/1 -> Data Type Conversion129/1
  Bitwise AND51/1 -> Shift Arithmetic38/1
  Bitwise AND50/1 -> Shift Arithmetic37/1
  Data Type Conversion2/1 -> Multiply/1
  Bitwise AND54/1 -> Shift Arithmetic40/1
  Bitwise AND55/1 -> Shift Arithmetic41/1
  Shift Arithmetic39/1 -> Data Type Conversion133/1
  Data Type Conversion131/1 -> Bitwise AND52/1, Bitwise AND53/1, Bitwise AND54/1, Bitwise AND55/1
  Bitwise AND53/1 -> Shift Arithmetic39/1
  Bitwise AND52/1 -> Data Type Conversion132/1
  Shift Arithmetic41/1 -> Data Type Conversion130/1
  Shift Arithmetic40/1 -> Data Type Conversion44/1
  Multiply1/1 -> Data Type Conversion131/1
  Data Type Conversion132/1 -> Mux/116
  Data Type Conversion133/1 -> Mux/117
  Data Type Conversion44/1 -> Mux/118
  Data Type Conversion130/1 -> Mux/119
  Data Type Conversion3/1 -> Multiply1/1
  VOUTP_HoodSW_flg/1 -> Data Type Conversion134/1
  VOUTP_TailgateHDSW_flg/1 -> Data Type Conversion137/1
  VOUTP_CTDLockSW_flg/1 -> Data Type Conversion136/1
  VOUTP_TailgateSW_flg/1 -> Data Type Conversion135/1
  VOUTP_APMDoorControlSta_flg/1 -> Data Type Conversion138/1
  Data Type Conversion138/1 -> Mux/124
  VHAL_funAuto_flg/1 -> Data Type Conversion139/1
  VHAL_DiagDRLOFF_flg/1 -> Data Type Conversion140/1
  Data Type Conversion139/1 -> Mux/125
  Data Type Conversion140/1 -> Mux/126
  Data Type Conversion141/1 -> Mux/127
  Data Type Conversion142/1 -> Mux/128
  Data Type Conversion143/1 -> Mux/129
  Data Type Conversion144/1 -> Mux/130
  Data Type Conversion145/1 -> Mux/131
  Demux/1 -> Data Type Conversion146/1
  Demux/2 -> Data Type Conversion147/1
  Demux/3 -> Data Type Conversion148/1
  Demux/4 -> Data Type Conversion149/1
  Demux/5 -> Data Type Conversion150/1
  Demux/6 -> Data Type Conversion151/1
  Demux/7 -> Data Type Conversion152/1
  Demux/8 -> Data Type Conversion153/1
  VHAL_USSConfig_raw8/1 -> Demux/1
  Data Type Conversion146/1 -> Mux/132
  Data Type Conversion147/1 -> Mux/133
  Data Type Conversion148/1 -> Mux/134
  Data Type Conversion149/1 -> Mux/135
  Data Type Conversion150/1 -> Mux/136
  Data Type Conversion151/1 -> Mux/137
  Data Type Conversion152/1 -> Mux/138
  Data Type Conversion153/1 -> Mux/139
  Demux/16 -> Data Type Conversion161/1
  Demux/15 -> Data Type Conversion160/1
  Demux/14 -> Data Type Conversion159/1
  Demux/13 -> Data Type Conversion158/1
  Demux/12 -> Data Type Conversion157/1
  Demux/11 -> Data Type Conversion156/1
  Demux/10 -> Data Type Conversion155/1
  Demux/9 -> Data Type Conversion154/1
  Data Type Conversion154/1 -> Mux/140
  Data Type Conversion155/1 -> Mux/141
  Data Type Conversion156/1 -> Mux/142
  Data Type Conversion157/1 -> Mux/143
  Data Type Conversion158/1 -> Mux/144
  Data Type Conversion159/1 -> Mux/145
  Data Type Conversion160/1 -> Mux/146
  Data Type Conversion161/1 -> Mux/147
  Data Type Conversion177/1 -> Mux/163
  Data Type Conversion176/1 -> Mux/162
  Data Type Conversion175/1 -> Mux/161
  Data Type Conversion174/1 -> Mux/160
  Data Type Conversion173/1 -> Mux/159
  Data Type Conversion172/1 -> Mux/158
  Data Type Conversion171/1 -> Mux/157
  Data Type Conversion170/1 -> Mux/156
  Demux1/9 -> Data Type Conversion170/1
  Demux1/10 -> Data Type Conversion171/1
  Demux1/11 -> Data Type Conversion172/1
  Demux1/12 -> Data Type Conversion173/1
  Demux1/13 -> Data Type Conversion174/1
  Demux1/14 -> Data Type Conversion175/1
  Demux1/15 -> Data Type Conversion176/1
  Demux1/16 -> Data Type Conversion177/1
  Data Type Conversion169/1 -> Mux/155
  Data Type Conversion168/1 -> Mux/154
  Data Type Conversion167/1 -> Mux/153
  Data Type Conversion166/1 -> Mux/152
  Data Type Conversion165/1 -> Mux/151
  Data Type Conversion164/1 -> Mux/150
  Data Type Conversion163/1 -> Mux/149
  Data Type Conversion162/1 -> Mux/148
  VHAL_TireSize_raw8/1 -> Demux1/1
  Demux1/8 -> Data Type Conversion169/1
  Demux1/7 -> Data Type Conversion168/1
  Demux1/6 -> Data Type Conversion167/1
  Demux1/5 -> Data Type Conversion166/1
  Demux1/4 -> Data Type Conversion165/1
  Demux1/3 -> Data Type Conversion164/1
  Demux1/2 -> Data Type Conversion163/1
  Demux1/1 -> Data Type Conversion162/1
  Demux2/1 -> Data Type Conversion178/1
  Demux2/2 -> Data Type Conversion179/1
  Demux2/3 -> Data Type Conversion180/1
  Demux2/4 -> Data Type Conversion181/1
  Demux2/5 -> Data Type Conversion182/1
  Demux2/6 -> Data Type Conversion183/1
  Demux2/7 -> Data Type Conversion184/1
  Demux2/8 -> Data Type Conversion185/1
  VHAL_APSFunConfig_raw8/1 -> Demux2/1
  Data Type Conversion178/1 -> Mux/164
  Data Type Conversion179/1 -> Mux/165
  Data Type Conversion180/1 -> Mux/166
  Data Type Conversion181/1 -> Mux/167
  Data Type Conversion182/1 -> Mux/168
  Data Type Conversion183/1 -> Mux/169
  Data Type Conversion184/1 -> Mux/170
  Data Type Conversion185/1 -> Mux/171
  Demux2/16 -> Data Type Conversion193/1
  Demux2/15 -> Data Type Conversion192/1
  Demux2/14 -> Data Type Conversion191/1
  Demux2/13 -> Data Type Conversion190/1
  Demux2/12 -> Data Type Conversion189/1
  Demux2/11 -> Data Type Conversion188/1
  Demux2/10 -> Data Type Conversion187/1
  Demux2/9 -> Data Type Conversion186/1
  Data Type Conversion186/1 -> Mux/172
  Data Type Conversion187/1 -> Mux/173
  Data Type Conversion188/1 -> Mux/174
  Data Type Conversion189/1 -> Mux/175
  Data Type Conversion190/1 -> Mux/176
  Data Type Conversion191/1 -> Mux/177
  Data Type Conversion192/1 -> Mux/178
  Data Type Conversion193/1 -> Mux/179
  VOUTP_fUnlockSingle_flg/1 -> Data Type Conversion194/1
  Data Type Conversion194/1 -> Mux/180
  Gain3/1 -> Data Type Conversion145/1
  Gain2/1 -> Data Type Conversion144/1
  Gain1/1 -> Data Type Conversion143/1
  Gain/1 -> Data Type Conversion142/1
  Subsystem/1(Out1) -> Data Type Conversion141/1
  VHAL_DiagFMHT_s/1 -> Subsystem/1(VOUTP_DiagFMHT_s)
  VHAL_DiagFRTC_mA/1 -> Gain1/1
  VHAL_DiagRLTC_mA/1 -> Gain2/1
  VHAL_DiagRRTC_mA/1 -> Gain3/1
  VHAL_DiagFLTC_mA/1 -> Gain/1
  VOUTP_SaveRegenMode_enum/1 -> Data Type Conversion195/1
  Data Type Conversion195/1 -> Mux/181
  Data Type Conversion212/1 -> Mux/198
  VOUTP_AmbPwrWarnENFlash_enum/1 -> Data Type Conversion200/1
  Data Type Conversion197/1 -> Mux/183
  Data Type Conversion199/1 -> Mux/185
  VOUTP_AmbColorSta5_enum/1 -> Data Type Conversion206/1
  VOUTP_AmbBrightnessSta1_enum/1 -> Data Type Conversion208/1
  VOUTP_AmbBrightnessSta3_enum/1 -> Data Type Conversion210/1
  Data Type Conversion213/1 -> Mux/199
  Data Type Conversion196/1 -> Mux/182
  Data Type Conversion202/1 -> Mux/188
  Data Type Conversion200/1 -> Mux/186
  VOUTP_AmbBrightnessSta2_enum/1 -> Data Type Conversion209/1
  Data Type Conversion209/1 -> Mux/195
  Data Type Conversion201/1 -> Mux/187
  VOUTP_AmbColorSta3_enum/1 -> Data Type Conversion204/1
  VOUTP_AmbColorSta1_enum/1 -> Data Type Conversion202/1
  VOUTP_AmbBrightnessSta7_enum/1 -> Data Type Conversion213/1
  VOUTP_AmbColorSta4_enum/1 -> Data Type Conversion205/1
  VOUTP_AmbODAENFlash_enum/1 -> Data Type Conversion201/1
  VOUTP_AmbLinkDriStaFlash_enum/1 -> Data Type Conversion199/1
  VOUTP_AmbFunENFlash_enum/1 -> Data Type Conversion196/1
  Data Type Conversion204/1 -> Mux/190
  Data Type Conversion203/1 -> Mux/189
  VOUTP_AmbDimENFlash_enum/1 -> Data Type Conversion198/1
  VOUTP_AmbColorSta2_enum/1 -> Data Type Conversion203/1
  VOUTP_AmbColorSta7_enum/1 -> Data Type Conversion207/1
  Data Type Conversion208/1 -> Mux/194
  VOUTP_AmbWelENFlash_enum/1 -> Data Type Conversion197/1
  Data Type Conversion205/1 -> Mux/191
  VOUTP_AmbBrightnessSta4_enum/1 -> Data Type Conversion211/1
  Data Type Conversion207/1 -> Mux/193
  Data Type Conversion211/1 -> Mux/197
  Data Type Conversion210/1 -> Mux/196
  Data Type Conversion206/1 -> Mux/192
  VOUTP_AmbBrightnessSta5_enum/1 -> Data Type Conversion212/1
  Data Type Conversion198/1 -> Mux/184

== system SWC_FDC_type/run_SWC_FDC_RxTx_5ms_sys/Subsystem2/DKC2/DKC Decryption and Unpack ==
  DKC_ResultData_16byte : Inport
  BHAL_CAN4_outputs : Inport  Port=2
  Enable : EnablePort
  Bitwise OR33 : simulink/Logic and Bit Operations/Bitwise Operator  logicop=OR  UseBitMask=off  NumInputPorts=4  BitMask=bin2dec('00000000000000000000')  BitMaskRealWorld=Stored Integer
  Bus Selector : BusSelector  OutputSignals=VHAL_PCommandToBCM_enum,VHAL_PCommandToPTG_enum,VHAL_PDKeyAreaLockUnlock_enum,VHAL_PDKeyAreaPS_enum,VHAL_PDKeyAreaPTG_enum
  Constant{1..4} (4 alike) : Constant  Commented=on  Value=0x04
  DKCReVehData : Subsystem  AncestorBlock=dkc2/DKC/Subsystem/VDKC_DKCDecryptionDATA_enum Unpack/DKCReVehData
  DKCRemotePW : Subsystem  AncestorBlock=dkc2/DKC/Subsystem/VDKC_DKCDecryptionDATA_enum Unpack/DKCRemotePW
  Data Type Conversion{16,38..47} (11 alike) : DataTypeConversion  OutDataTypeStr=uint8
  Data Type Conversion36 : DataTypeConversion  OutDataTypeStr=boolean
  Data Type Conversion37 : DataTypeConversion  OutDataTypeStr=boolean
  Data Type Conversion{58,60..61,81,94} (5 alike) : DataTypeConversion  OutDataTypeStr=uint32
  Data Type Conversion{67..74} (8 alike) : DataTypeConversion  Commented=on  OutDataTypeStr=uint8
  Demux : Demux  Outputs=16
  Equal{,1..4} (5 alike) : RelationalOperator  Operator=~=  OutDataTypeStr=boolean  RndMeth=Simplest
  From6 : From  Commented=on  GotoTag=Byte_12
  From7 : From  Commented=on  GotoTag=Byte_13
  From8 : From  Commented=on  GotoTag=Byte_14
  From9 : From  Commented=on  GotoTag=Byte_15
  Logical Operator : Logic  Operator=OR  Inputs=5  AllPortsSameDT=off  OutDataTypeStr=boolean
  PCommandToBCM : Subsystem  AncestorBlock=dkc2/DKC/Subsystem/VDKC_DKCDecryptionDATA_enum Unpack/PCommandToBCM
  PCommandToPTG : Subsystem  AncestorBlock=dkc2/DKC/Subsystem/VDKC_DKCDecryptionDATA_enum Unpack/PCommandToPTG
  PDKeyAreaLockUnlock : Subsystem  AncestorBlock=dkc2/DKC/Subsystem/VDKC_DKCDecryptionDATA_enum Unpack/PDKeyAreaLockUnlock
  PDKeyAreaPS : Subsystem  AncestorBlock=dkc2/DKC/Subsystem/VDKC_DKCDecryptionDATA_enum Unpack/PDKeyAreaPS
  PDKeyAreaPTG : Subsystem  AncestorBlock=dkc2/DKC/Subsystem/VDKC_DKCDecryptionDATA_enum Unpack/PDKeyAreaPTG
  PDKeyWelcome : Subsystem  AncestorBlock=dkc2/DKC/Subsystem/VDKC_DKCDecryptionDATA_enum Unpack/PDKeyWelcome
  PDkeyShowIVI : Subsystem  AncestorBlock=dkc2/DKC/Subsystem/VDKC_DKCDecryptionDATA_enum Unpack/PDkeyShowIVI
  PKeyMiss : Subsystem  AncestorBlock=dkc2/DKC/Subsystem/VDKC_DKCDecryptionDATA_enum Unpack/PKeyMiss
  PKeyMode : Subsystem  AncestorBlock=dkc2/DKC/Subsystem/VDKC_DKCDecryptionDATA_enum Unpack/PKeyMode
  PUIDLowPower : Subsystem  AncestorBlock=dkc2/DKC/Subsystem/VDKC_DKCDecryptionDATA_enum Unpack/PUIDLowPower
  Shift Arithmetic33 : ArithShift  BitShiftNumber=8  BitShiftDirection=Left
  Shift Arithmetic34 : ArithShift  BitShiftNumber=16  BitShiftDirection=Left
  Shift Arithmetic35 : ArithShift  BitShiftNumber=24  BitShiftDirection=Left
  VHAL_DKCDecReVehData_enum : Outport
  VHAL_DKCDecRemotePW_enum : Outport  Port=2
  VHAL_DKCDecPCommandToBCM_enum : Outport  Port=3
  VHAL_DKCDecPCommandToPTG_enum : Outport  Port=4
  VHAL_DKCDecPDKeyAreaLockUnlock_enum : Outport  Port=5
  VHAL_DKCDecPDKeyAreaPS_enum : Outport  Port=6
  VHAL_DKCDecPDKeyAreaPTG_enum : Outport  Port=7
  VHAL_DKCDecPDKeyWelcome_enum : Outport  Port=8
  VHAL_DKCDecPDkeyShowIVI_enum : Outport  Port=9
  VHAL_DKCDecPKeyMiss_flg : Outport  Port=10
  VHAL_DKCDecPKeyMode_enum : Outport  Port=11
  VHAL_DKCDecPUIDLowPower_flg : Outport  Port=12
  VHAL_TimeSNDKCFbk_cnt : Outport  Port=13
  VHAL_DKCDecryptionFail_flg : Outport  Port=14
  wires:
  PDkeyShowIVI/1(VHAL_PDkeyShowIVI_enum) -> Data Type Conversion40/1
  PDKeyAreaLockUnlock/1(VHAL_PDKeyAreaLockUnlock_enum) -> Data Type Conversion45/1
  [Byte_0] -> PDKeyWelcome/1(Byte_0)
  DKCReVehData/1(VHAL_DKCReVehData_enum) -> Data Type Conversion39/1
  [Byte_3] -> PDKeyAreaPTG/1(Byte_3)
  Demux/2 -> [Byte_1]
  PCommandToBCM/1(VHAL_PCommandToBCM_enum) -> Data Type Conversion47/1
  Data Type Conversion44/1 -> [VHAL_DKCDecPDKeyAreaPS_enum], VHAL_DKCDecPDKeyAreaPS_enum/1
  [Byte_3] -> DKCRemotePW/1(Byte_3)
  PDKeyAreaPTG/1(VHAL_PDKeyAreaPTG_enum) -> Data Type Conversion43/1
  Demux/5 -> [Byte_4]
  Demux/3 -> [Byte_2]
  PDKeyWelcome/1(VHAL_PDKeyWelcome_enum) -> Data Type Conversion42/1
  Demux/6 -> [Byte_5]
  [Byte_3] -> PKeyMiss/1(Byte_3)
  Demux/7 -> [Byte_6]
  DKCRemotePW/1(VHAL_DKCRemotePW_enum) -> Data Type Conversion38/1
  Demux/8 -> [Byte_7]
  Data Type Conversion40/1 -> VHAL_DKCDecPDkeyShowIVI_enum/1
  Demux/9 -> [Byte_8]
  Data Type Conversion42/1 -> VHAL_DKCDecPDKeyWelcome_enum/1
  Demux/10 -> [Byte_9]
  Demux/1 -> [Byte_0]
  [Byte_11] -> Data Type Conversion81/1
  Demux/11 -> [Byte_10]
  PKeyMode/1(VHAL_PKeyMode_enum) -> Data Type Conversion41/1
  Data Type Conversion43/1 -> [VHAL_DKCDecPDKeyAreaPTG_enum], VHAL_DKCDecPDKeyAreaPTG_enum/1
  Data Type Conversion94/1 -> VHAL_TimeSNDKCFbk_cnt/1
  PUIDLowPower/1(VHAL_PUIDLowPower_flg) -> Data Type Conversion37/1
  Data Type Conversion41/1 -> VHAL_DKCDecPKeyMode_enum/1
  Data Type Conversion45/1 -> [VHAL_DKCDecPDKeyAreaLockUnlock_enum], VHAL_DKCDecPDKeyAreaLockUnlock_enum/1
  [Byte_0] -> PCommandToBCM/1(Byte_0)
  PCommandToPTG/1(VHAL_PCommandToPTG_enum) -> Data Type Conversion46/1
  Data Type Conversion37/1 -> VHAL_DKCDecPUIDLowPower_flg/1
  [Byte_1] -> PDKeyAreaPS/1(Byte_1)
  [Byte_2] -> PDkeyShowIVI/1(Byte_2)
  [Byte_1] -> PDKeyAreaLockUnlock/1(Byte_1)
  Bitwise OR33/1 -> Data Type Conversion94/1
  Shift Arithmetic35/1 -> Bitwise OR33/1
  [Byte_1] -> PUIDLowPower/1(Byte_1)
  PDKeyAreaPS/1(VHAL_PDKeyAreaPS_enum) -> Data Type Conversion44/1
  Data Type Conversion58/1 -> Shift Arithmetic35/1
  Data Type Conversion60/1 -> Shift Arithmetic34/1
  Data Type Conversion46/1 -> [VHAL_DKCDecPCommandToPTG_enum], VHAL_DKCDecPCommandToPTG_enum/1
  Shift Arithmetic34/1 -> Bitwise OR33/2
  Shift Arithmetic33/1 -> Bitwise OR33/3
  Data Type Conversion36/1 -> VHAL_DKCDecPKeyMiss_flg/1
  PKeyMiss/1(VHAL_PKeyMiss_flg) -> Data Type Conversion36/1
  [Byte_8] -> Data Type Conversion58/1
  [Byte_2] -> PKeyMode/1(Byte_2)
  Data Type Conversion38/1 -> VHAL_DKCDecRemotePW_enum/1
  [Byte_4] -> DKCReVehData/1(Byte_4)
  Data Type Conversion61/1 -> Shift Arithmetic33/1
  [Byte_10] -> Data Type Conversion61/1
  [Byte_9] -> Data Type Conversion60/1
  [Byte_1] -> PCommandToPTG/1(Byte_1)
  Data Type Conversion47/1 -> [VHAL_DKCDecPCommandToBCM_enum], VHAL_DKCDecPCommandToBCM_enum/1
  Demux/12 -> [Byte_11]
  Data Type Conversion81/1 -> Bitwise OR33/4
  Data Type Conversion39/1 -> VHAL_DKCDecReVehData_enum/1
  Demux/4 -> [Byte_3]
  Data Type Conversion16/1 -> Demux/1  "VHAL_DKCResultData_raw"
  DKC_ResultData_16byte/1 -> Data Type Conversion16/1
  Demux/14 -> [Byte_13]
  Demux/15 -> [Byte_14]
  Demux/16 -> [Byte_15]
  Demux/13 -> [Byte_12]
  Constant1/1 -> Data Type Conversion68/1
  Equal3/1 -> Logical Operator/4
  Constant2/1 -> Data Type Conversion70/1
  From6/1 -> Data Type Conversion67/1
  Equal1/1 -> Logical Operator/2
  Equal/1 -> Logical Operator/1
  From8/1 -> Data Type Conversion71/1
  Constant4/1 -> Data Type Conversion74/1
  Equal2/1 -> Logical Operator/3
  From9/1 -> Data Type Conversion73/1
  Constant3/1 -> Data Type Conversion72/1
  Logical Operator/1 -> VHAL_DKCDecryptionFail_flg/1
  From7/1 -> Data Type Conversion69/1
  BHAL_CAN4_outputs/1 -> Bus Selector/1
  [VHAL_DKCDecPCommandToBCM_enum] -> Equal/1
  [VHAL_DKCDecPCommandToPTG_enum] -> Equal1/1
  [VHAL_DKCDecPDKeyAreaLockUnlock_enum] -> Equal2/1
  [VHAL_DKCDecPDKeyAreaPS_enum] -> Equal3/1
  Bus Selector/1 -> Equal/2  "<VHAL_PCommandToBCM_enum>"
  Bus Selector/2 -> Equal1/2  "<VHAL_PCommandToPTG_enum>"
  Bus Selector/3 -> Equal2/2  "<VHAL_PDKeyAreaLockUnlock_enum>"
  Bus Selector/4 -> Equal3/2  "<VHAL_PDKeyAreaPS_enum>"
  [VHAL_DKCDecPDKeyAreaPTG_enum] -> Equal4/1
  Bus Selector/5 -> Equal4/2  "<VHAL_PDKeyAreaPTG_enum>"
  Equal4/1 -> Logical Operator/5

== system SWC_FDC_type/run_SWC_FDC_RxTx_5ms_sys/Halin_CDD/Halin_TPMS/Subsystem/CRC8_Caculation ==
  MsgData : Inport
  Data Type Conversion1 : DataTypeConversion  OutDataTypeStr=uint16
  Data Type Conversion2 : DataTypeConversion  OutDataTypeStr=uint8
  MATLAB Function : MATLAB Function  TreatAsAtomicUnit=on
  CRCout : Outport
  wires:
  Data Type Conversion1/1 -> MATLAB Function/1(msg_raw)
  MATLAB Function/1(CRC_Out) -> Data Type Conversion2/1
  MsgData/1 -> Data Type Conversion1/1
  Data Type Conversion2/1 -> CRCout/1
